simulink model "nonLinearModel"  (R2014b)
settings: Solver=ode4  SolverMode=SingleTasking  StartTime=0.0  StopTime=TIME_SIM  FixedStep=STEP_SIZE  RelTol=1e-3
values from neighbouring files (symbols this model uses):
  b1 = 2.6826    [main.m]    (also in mainbis.m)
  b2 = -4.0269*10^3    (= -4026.9)    [main.m]    (also in mainbis.m)
  Bl0 = 14.54    [main.m]    (also in mainbis.m)
  k0 = 6259.3    [main.m]    (also in mainbis.m)
  k1 = -1.4562*10^5    (= -145620)    [main.m]    (also in mainbis.m)
  k2 = 2.6106*10^7    (= 26106000)    [main.m]    (also in mainbis.m)
  l1 = -5.2937*10^(-1)    (= -0.52937)    [main.m]    (also in mainbis.m)
  l2 = -1.2012*10^2    (= -120.12)    [main.m]    (also in mainbis.m)
  Le0 = 5.65*10^(-3)    (= 0.00565)    [main.m]    (also in mainbis.m)
  mt = 52.08*10^(-3)    (= 0.05208)    [main.m]    (also in mainbis.m)
  Re = 7.9    [main.m]    (also in mainbis.m)
  Rm = 2.628    [main.m]    (also in mainbis.m)
settings Model: Creator=Kate  LastModifiedBy=Kate

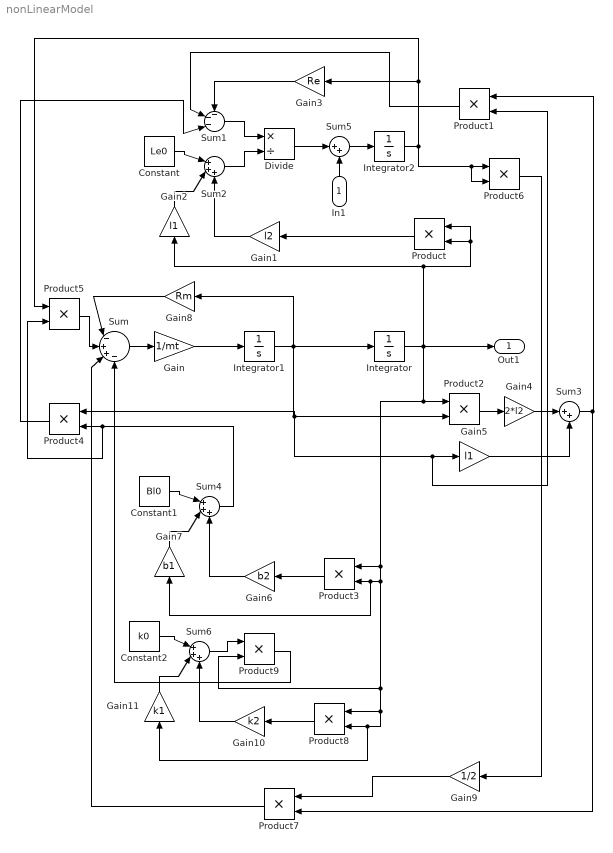
== system nonLinearModel ==
  In1 : Inport
  Constant : Constant  Value=Le0
  Constant1 : Constant  Value=Bl0
  Constant2 : Constant  Value=k0
  Divide : Product  Inputs=*/
  Gain : Gain  Gain=1/mt
  Gain1 : Gain  Gain=l2
  Gain10 : Gain  Gain=k2
  Gain11 : Gain  Gain=k1
  Gain2 : Gain  Gain=l1
  Gain3 : Gain  Gain=Re
  Gain4 : Gain  Gain=2*l2
  Gain5 : Gain  Gain=l1
  Gain6 : Gain  Gain=b2
  Gain7 : Gain  Gain=b1
  Gain8 : Gain  Gain=Rm
  Gain9 : Gain  Gain=1/2
  Integrator : Integrator
  Integrator1 : Integrator
  Integrator2 : Integrator
  Product{,1..9} (10 alike) : Product
  Sum : Sum  Inputs=|-++-
  Sum1 : Sum  Inputs=---|
  Sum2 : Sum  Inputs=|+++
  Sum3 : Sum  Inputs=|++
  Sum4 : Sum  Inputs=|+++
  Sum5 : Sum  Inputs=|++
  Sum6 : Sum  Inputs=|+++
  Out1 : Outport
  wires:
  Integrator1/1 -> Gain8/1, Product1/2, Gain5/1, Product4/1, Product2/2, Integrator/1
  Sum/1 -> Gain/1
  Gain/1 -> Integrator1/1
  Sum1/1 -> Divide/1
  Sum2/1 -> Divide/2
  Integrator/1 -> Product9/2, Gain11/1, Product8/2, Product8/1, Gain7/1, Product3/2, Product3/1, Product2/1, Gain2/1, Product/1, Product/2, Out1/1
  Constant/1 -> Sum2/1
  Product/1 -> Gain1/1
  Gain1/1 -> Sum2/3
  Gain2/1 -> Sum2/2
  Integrator2/1 -> Product6/2, Product6/1, Product5/1, Gain3/1
  Gain3/1 -> Sum1/1
  Product2/1 -> Gain4/1
  Gain4/1 -> Sum3/1
  Gain5/1 -> Sum3/2
  Sum3/1 -> Product7/2, Product1/1
  Product1/1 -> Sum1/2
  Constant1/1 -> Sum4/1
  Product3/1 -> Gain6/1
  Gain6/1 -> Sum4/3
  Gain7/1 -> Sum4/2
  Sum4/1 -> Product5/2, Product4/2
  Product4/1 -> Sum1/3
  Sum5/1 -> Integrator2/1
  Divide/1 -> Sum5/1
  In1/1 -> Sum5/2
  Product5/1 -> Sum/2
  Gain8/1 -> Sum/1
  Gain9/1 -> Product7/1
  Product6/1 -> Gain9/1
  Product7/1 -> Sum/3
  Product8/1 -> Gain10/1
  Gain10/1 -> Sum6/3
  Gain11/1 -> Sum6/2
  Constant2/1 -> Sum6/1
  Sum6/1 -> Product9/1
  Product9/1 -> Sum/4
